simulink model "closed_loop"  (R2023a)
settings: Solver=FixedStepAuto  StartTime=0.0  StopTime=10  FixedStep=1/1000  RelTol=1e-3  AbsTol=1e-3
model workspace: external: MATLAB File params.m (data not in the file)
values from neighbouring files (symbols this model uses):
  g = 9.81    [Linearization.m]    (also in params.m)
  m = 0.027    [Linearization.m]    (also in params.m)
libraries: nesl_utility x9
settings Model: Creator=Jocke  LastModifiedBy=mosta
settings SolverCC: AutoScaleAbsTol=off  AlgebraicLoopSolver=TrustRegion
settings DataIOCC: ReturnWorkspaceOutputs=off
settings OptimizationCC: UseDivisionForNetSlopeComputation=on
settings DebuggingCC: UnconnectedInputMsg=warning  UnconnectedOutputMsg=warning  UnconnectedLineMsg=warning  ArithmeticOperatorsInVariantConditions=warning
settings ModelReferenceCC: EnableRefExpFcnMdlSchedulingChecks=on
settings SFSimCC: SimUseLocalCustomCode=off  CustomCodeUndefinedFunction=UseInterfaceOnly
settings RTWCC: RTWUseLocalCustomCode=off  Toolchain=GNU gcc/g++ | gmake (64-bit Linux)
settings CodeAppCC: StateflowObjectComments=on
settings SimscapeCC: SimscapeNormalizeSystem=off  SimscapeLogType=all  SimscapeLogDataHistory=10000

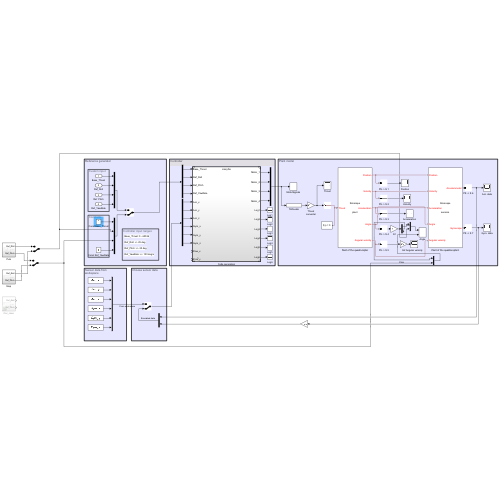
[thumbnail: Simulink's stored preview of the top-level diagram]
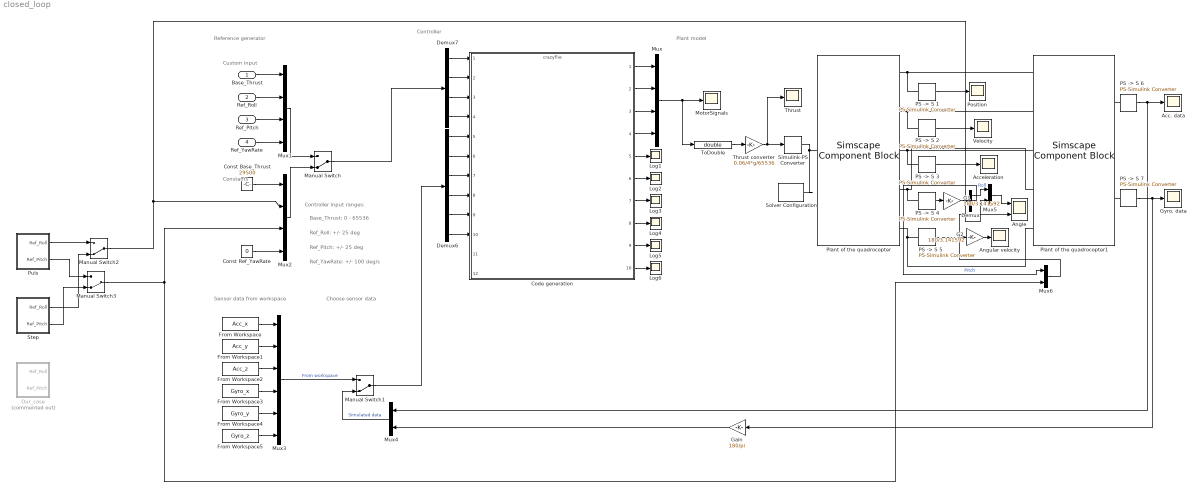
== system closed_loop ==
  note: Custom input
  note: Plant model
  note: Controller
  note: Constants
  note: Reference generator
  note: Ref_Roll: +/- 25 deg
  note: Base_Thrust: 0 - 65536
  note: Ref_Pitch: +/- 25 deg
  note: Ref_YawRate: +/- 100 deg/s
  note: Controller input ranges:
  note: Sensor data from
      | workspace
  note: Choose sensor data
  Base_Thrust : Inport  OutDataTypeStr=double
  Ref_Roll : Inport  Port=2  OutDataTypeStr=double
  Ref_Pitch : Inport  Port=3  OutDataTypeStr=double
  Ref_YawRate : Inport  Port=4  OutDataTypeStr=double
  Acc. data : Scope
  Acceleration : Scope
  Angle : Scope  NumInputPorts=2
  Angular velocity : Scope
  Code generation : ModelReference  ModelNameDialog=crazyflie.slx  SimulationMode=Normal  ModelReferenceVersion=8.0
  Const Base_Thrust : Constant  Value=29500
  Const Ref_YawRate : Constant  Value=0
  Demux : Demux  Outputs=3
  Demux6 : Demux  Outputs=6
  Demux7 : Demux
  From Workspace : FromWorkspace  VariableName=Acc_x  OutDataTypeStr=double
  From Workspace1 : FromWorkspace  VariableName=Acc_y  OutDataTypeStr=double
  From Workspace2 : FromWorkspace  VariableName=Acc_z  OutDataTypeStr=double
  From Workspace3 : FromWorkspace  VariableName=Gyro_x  OutDataTypeStr=double
  From Workspace4 : FromWorkspace  VariableName=Gyro_y  OutDataTypeStr=double
  From Workspace5 : FromWorkspace  VariableName=Gyro_z  OutDataTypeStr=double
  G1 : Gain  Gain=180/3.141592
  G2 : Gain  Gain=180/3.141592
  Gain : Gain  Gain=180/pi
  Gyro. data : Scope
  Log{1..6} (6 alike) : Scope
  Manual Switch{,1..3} (4 alike) : ManualSwitch  CurrentSetting=0
  MotorSignals : Scope
  Mux : Mux
  Mux1 : Mux
  Mux2 : Mux
  Mux3 : Mux  Inputs=6
  Mux4 : Mux  Inputs=2
  Mux5 : Mux  Inputs=2
  Mux6 : Mux  Inputs=2
  Our_case : Subsystem  Commented=on
  PS -> S {1..7} (7 alike) : nesl_utility/PS-Simulink Converter  PhysicalDomain=network_engine_domain  SubClassName=ps_output  LeftPortType=input  RightPortType=output  PseudoPeriodic=off  Frequencies=[]  VectorFormat=1-D array  Unit=1  AffineConversion=off
  Plant of the quadrocopter : SimscapeComponentBlock  SourceFile=plant  ComponentPath=plant  ComponentVariants=plant  ComponentVariantNames=plant  ClassName=plant  SchemaVersion=1  m=m kg  g=g m/s^2  d=d m  lift=lift N*s^2/rad^2  drag=drag N*m/(rad/s)^2  F=0.25 N*s/m  c=0 m/s^2
      settings: CopyFcn=simscape.engine.sli.internal.componentblockcallback(gcbh,'COPY')  PreCopyFcn=simscape.engine.sli.internal.componentblockcallback(gcbh,'PRECOPY')  PreDeleteFcn=simscape.engine.sli.internal.componentblockcallback(gcbh,'PREDELETE')  InternalSimscapePortConfiguration="{\"Bottom\":[],\"Left\":[{\"id\":\"ctrl\",\"label\":\"Thrust\",\"type\":\"input\"}],\"Right\":[{\"id\":\"pos\",\"label\":\"Position\",\"type\":\"output\"},{\"id\":\"v\",\"label\":\"Velocity\",\"type\":\"output\"},{\"id\":\"a\",\"label\":\"Acceleration\",\"type\":\"output\"},{\"id\":\"angle\",\"label\":\"Angle\",\"type\":\"output\"},{\"id\":\"w\",\"label\":\"Angular velocity\",\"type\":\"output\"}],\"Top\":[]}"
      mask Type: Plant of quadrocopter
  Plant of the quadrocopter1 : SimscapeComponentBlock  SourceFile=sensors  ComponentPath=sensors  ComponentVariants=sensors  ComponentVariantNames=sensors  ClassName=sensors  SchemaVersion=1  m=0.027 kg  g=9.81 m/s^2  d=0.046 m  k=2.5383e-11 m  b=1.9796e-9
      settings: CopyFcn=simscape.engine.sli.internal.componentblockcallback(gcbh,'COPY')  PreCopyFcn=simscape.engine.sli.internal.componentblockcallback(gcbh,'PRECOPY')  PreDeleteFcn=simscape.engine.sli.internal.componentblockcallback(gcbh,'PREDELETE')  InternalSimscapePortConfiguration="{\"Bottom\":[],\"Left\":[{\"id\":\"pos\",\"label\":\"Position\",\"type\":\"input\"},{\"id\":\"v\",\"label\":\"Velocity\",\"type\":\"input\"},{\"id\":\"a\",\"label\":\"Acceleration\",\"type\":\"input\"},{\"id\":\"angle\",\"label\":\"Angle\",\"type\":\"input\"},{\"id\":\"w\",\"label\":\"Angular velocity\",\"type\":\"input\"}],\"Right\":[{\"id\":\"acc\",\"label\":\"Accelerometer\",\"type\":\"output\"},{\"id\":\"gyro\",\"label\":\"Gyroscope\",\"type\":\"output\"}],\"Top\":[]}"
      mask Type: Plant of quadrocopter
  Position : Scope
  Puls : Subsystem
  Simulink-PS Converter : nesl_utility/Simulink-PS Converter  PhysicalDomain=network_engine_domain  SubClassName=ps_input  LeftPortType=input  RightPortType=output  PseudoPeriodic=off  Frequencies=[]  NoiseDistribution=none  NoiseParameters=[]  Unit=1  AffineConversion=off  FilteringAndDerivatives=zero  SimscapeFilterOrder=1  InputFilterTimeConstant=0.001  UdotUserProvided=1
  Solver Configuration : nesl_utility/Solver Configuration  PhysicalDomain=network_engine_domain  SubClassName=solver  LeftPortType=input  RightPortType=generic  Tones=[]  Harmonics=[]  SimulateNoise=off  Profile=off  UseLocalSampling=off  EnableSwitchedLinearOptims=on  FrequencyDomain=off  UseCCode=off  RelTol=0.001  AbsTol=1e-06  MinStep=1e-09  ToWorkspace=off  RevertToSquareIcSolve=off  NumHomotopyIterations=100  PhasorMode=off  PhasorModeNumHarmonics=1  ConsistencySolver=NEWTON_FTOL  IndexReductionMethod=DerivativeReplacement  DoDC=off  ResidualTolerance=1e-09  ConsistencyTolSource=GLOBAL  ConsistencyAbsTol=0.001  ConsistencyRelTol=0.001  ConsistencyTolFactor=0.001  UseLocalSolver=off  LocalSolverChoice=NE_BACKWARD_EULER_ADVANCER  ResolveIndetEquations=on  FunctionEvalNumThread=1  LocalSolverSampleTime=0.001  DoFixedCost=off  MaxNonlinIter=3  MaxModeIter=2  ComputeImpulses=off  ImpulseIterations=2  LinearAlgebra=Sparse  LinearAlgebraNumThread=0  EquationFormulation=NE_TIME_EF  DelaysMemoryBudget=1024  AutomaticFiltering=on  FilteringTimeConstant=0.001  PartitionStorageMethod=AS_NEEDED  PartitionMemoryBudget=1024  PartitionMethod=FAST
  Step : Subsystem
  Thrust : Scope
  Thrust converter : Gain  Gain=0.06/4*g/65536
  ToDouble : DataTypeConversion  OutDataTypeStr=double  RndMeth=Round
  Velocity : Scope
  wires:
  Code generation/1 -> Mux/1
  Code generation/4 -> Mux/4
  Code generation/3 -> Mux/3
  Code generation/2 -> Mux/2
  "PS -> S 7"/1 -> Gain/1, Gyro. data/1
  Code generation/5 -> Log1/1
  Code generation/6 -> Log2/1
  Code generation/7 -> Log3/1
  Code generation/8 -> Log4/1
  Code generation/9 -> Log5/1
  Code generation/10 -> Log6/1
  Mux/1 -> MotorSignals/1, ToDouble/1
  Base_Thrust/1 -> Mux1/1
  Ref_Roll/1 -> Mux1/2
  Ref_Pitch/1 -> Mux1/3
  Ref_YawRate/1 -> Mux1/4
  Mux1/1 -> Manual Switch/1
  Const Base_Thrust/1 -> Mux2/1
  Const Ref_YawRate/1 -> Mux2/4
  Mux2/1 -> Manual Switch/2
  Manual Switch/1 -> Demux7/1
  Demux7/1 -> Code generation/1
  Demux7/2 -> Code generation/2
  Demux7/3 -> Code generation/3
  Demux7/4 -> Code generation/4
  G2/1 -> Angular velocity/1
  ToDouble/1 -> Thrust converter/1
  Thrust converter/1 -> Thrust/1, Simulink-PS Converter/1
  "PS -> S 1"/1 -> Position/1
  "PS -> S 5"/1 -> G2/1
  "PS -> S 3"/1 -> Acceleration/1
  "PS -> S 2"/1 -> Velocity/1
  From Workspace5/1 -> Mux3/6
  From Workspace4/1 -> Mux3/5
  From Workspace3/1 -> Mux3/4
  From Workspace2/1 -> Mux3/3
  From Workspace1/1 -> Mux3/2
  From Workspace/1 -> Mux3/1
  Mux3/1 -> Manual Switch1/1  "From workspace"
  Demux6/1 -> Code generation/5
  Demux6/2 -> Code generation/6
  Demux6/3 -> Code generation/7
  Demux6/4 -> Code generation/8
  Demux6/5 -> Code generation/9
  Demux6/6 -> Code generation/10
  Manual Switch1/1 -> Demux6/1
  Mux4/1 -> Manual Switch1/2  "Simulated data"
  Demux/1 -> Mux5/1  "Roll"
  Demux/2 -> Mux6/1  "Pitch"
  G1/1 -> Demux/1
  "PS -> S 4"/1 -> G1/1
  Mux5/1 -> Angle/1
  Mux6/1 -> Angle/2
  "PS -> S 6"/1 -> Mux4/1, Acc. data/1
  Gain/1 -> Mux4/2
  Puls/1(Ref_Roll) -> Manual Switch2/1
  Manual Switch2/1 -> Mux5/2, Mux2/2
  Manual Switch3/1 -> Mux2/3, Mux6/2
  Puls/2(Ref_Pitch) -> Manual Switch3/1
  Step/1(Ref_Roll) -> Manual Switch2/2
  Step/2(Ref_Pitch) -> Manual Switch3/2
  connections:
  Simulink-PS Converter/RConn1 -- Solver Configuration/RConn1 -- Plant of the quadrocopter/LConn1
  Plant of the quadrocopter1/LConn1 -- "PS -> S 1"/LConn1 -- Plant of the quadrocopter/RConn1
  Plant of the quadrocopter1/LConn2 -- "PS -> S 2"/LConn1 -- Plant of the quadrocopter/RConn2
  Plant of the quadrocopter1/LConn3 -- "PS -> S 3"/LConn1 -- Plant of the quadrocopter/RConn3
  Plant of the quadrocopter1/LConn4 -- "PS -> S 4"/LConn1 -- Plant of the quadrocopter/RConn4
  Plant of the quadrocopter1/LConn5 -- Plant of the quadrocopter/RConn5 -- "PS -> S 5"/LConn1
  Plant of the quadrocopter1/RConn1 -- "PS -> S 6"/LConn1
  Plant of the quadrocopter1/RConn2 -- "PS -> S 7"/LConn1

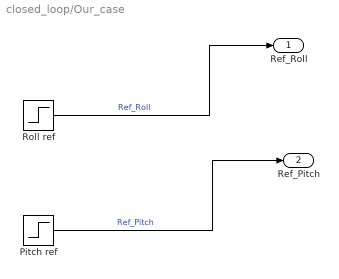
== system closed_loop/Our_case ==
  Pitch ref : Step  Time=6  After=5  SampleTime=0
  Roll ref : Step  Time=6  After=10  SampleTime=0
  Ref_Roll : Outport
  Ref_Pitch : Outport  Port=2
  wires:
  Roll ref/1 -> Ref_Roll/1  "Ref_Roll"
  Pitch ref/1 -> Ref_Pitch/1  "Ref_Pitch"

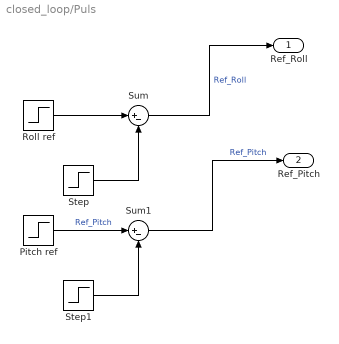
== system closed_loop/Puls ==
  Pitch ref : Step  Time=6  After=6  SampleTime=0
  Roll ref : Step  Time=4  After=6  SampleTime=0
  Step : Step  Time=4.1  After=6  SampleTime=0
  Step1 : Step  Time=6.1  After=6  SampleTime=0
  Sum : Sum  Inputs=|+-
  Sum1 : Sum  Inputs=|+-
  Ref_Roll : Outport
  Ref_Pitch : Outport  Port=2
  wires:
  Sum/1 -> Ref_Roll/1  "Ref_Roll"
  Roll ref/1 -> Sum/1
  Pitch ref/1 -> Sum1/1  "Ref_Pitch"
  Sum1/1 -> Ref_Pitch/1  "Ref_Pitch"
  Step/1 -> Sum/2
  Step1/1 -> Sum1/2

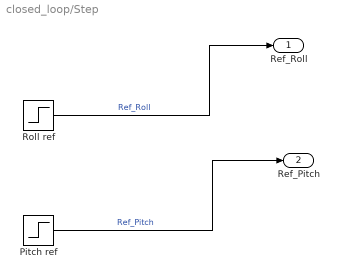
== system closed_loop/Step ==
  Pitch ref : Step  Time=4  After=10  SampleTime=0
  Roll ref : Step  Time=6  Before=10  After=0  SampleTime=0
  Ref_Roll : Outport
  Ref_Pitch : Outport  Port=2
  wires:
  Roll ref/1 -> Ref_Roll/1  "Ref_Roll"
  Pitch ref/1 -> Ref_Pitch/1  "Ref_Pitch"
